simulink model "linmodel_eq1_discr_lqr"  (R2019a)
settings: Solver=VariableStepAuto  StartTime=0.0  StopTime=30  RelTol=1e-3
InitFcn:
  | lin_discr_model
undefined symbols (not defined in the file): A_eq1_d, B_eq1_d, C_eq1_d, K122, L, Ts
settings Model: Creator=jessi  LastModifiedBy=jessi

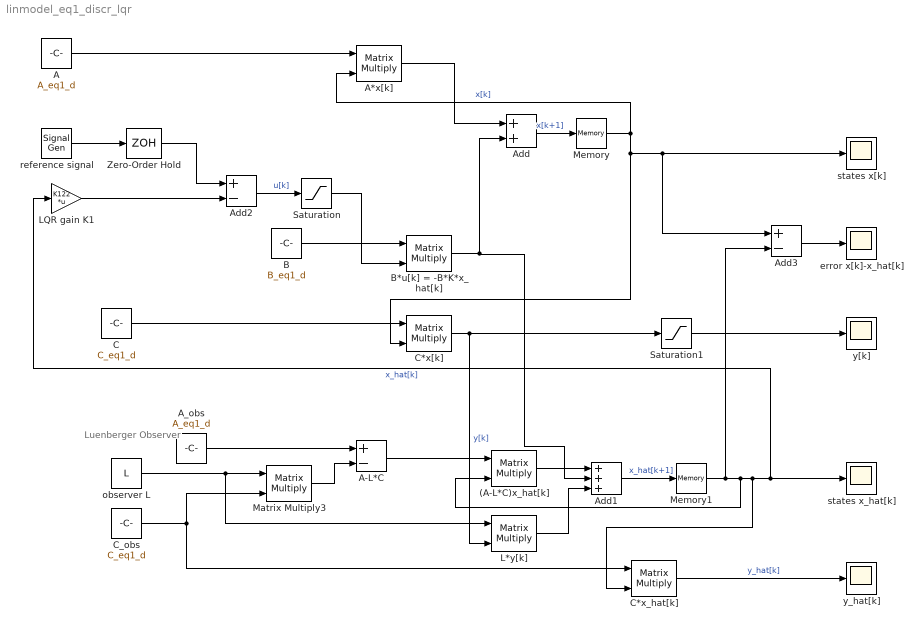
== system linmodel_eq1_discr_lqr ==
  note: Luenberger Observer
  (A-L*C)x_hat[k] : Product  Multiplication=Matrix(*)
  A : Constant  Value=A_eq1_d  SampleTime=Ts
  A*x[k] : Product  Multiplication=Matrix(*)
  A-L*C : Sum  Inputs=+-
  A_obs : Constant  Value=A_eq1_d
  Add : Sum
  Add1 : Sum  Inputs=+++
  Add2 : Sum  Inputs=+-
  Add3 : Sum  Inputs=+-
  B : Constant  Value=B_eq1_d  SampleTime=Ts
  B*u[k] = -B*K*x_hat[k] : Product  Multiplication=Matrix(*)
  C : Constant  Value=C_eq1_d  SampleTime=Ts
  C*x[k] : Product  Multiplication=Matrix(*)
  C*x_hat[k] : Product  Multiplication=Matrix(*)
  C_obs : Constant  Value=C_eq1_d
  L*y[k] : Product  Multiplication=Matrix(*)
  LQR gain K1 : Gain  Gain=K122  Multiplication=Matrix(K*u)
  Matrix Multiply3 : Product  Multiplication=Matrix(*)
  Memory : Memory  InitialCondition=[pi;0;0;0]
  Memory1 : Memory  InitialCondition=[pi; 0;0;0]
  Saturation : Saturate  UpperLimit=1  LowerLimit=-1
  Saturation1 : Saturate  UpperLimit=2*pi  LowerLimit=-2*pi
  Zero-Order Hold : ZeroOrderHold  SampleTime=Ts
  error x[k]-x_hat[k] : Scope
  observer L : Constant  Value=L  SampleTime=Ts
  reference signal : SignalGenerator  WaveForm=square  Amplitude=-0.3
  states x[k] : Scope
  states x_hat[k] : Scope
  y[k] : Scope
  y_hat[k] : Scope
  wires:
  B/1 -> B*u[k] = -B*K*x_hat[k]/1
  A/1 -> A*x[k]/1
  A*x[k]/1 -> Add/1
  B*u[k] = -B*K*x_hat[k]/1 -> Add1/2, Add/2
  Memory/1 -> A*x[k]/2, Add3/1, states x[k]/1, C*x[k]/2  "x[k]"
  C/1 -> C*x[k]/1
  C*x[k]/1 -> L*y[k]/2, Saturation1/1  "y[k]"
  observer L/1 -> L*y[k]/1, Matrix Multiply3/1
  Matrix Multiply3/1 -> A-L*C/2
  A-L*C/1 -> (A-L*C)x_hat[k]/1
  (A-L*C)x_hat[k]/1 -> Add1/1
  L*y[k]/1 -> Add1/3
  Add1/1 -> Memory1/1  "x_hat[k+1]"
  Memory1/1 -> Add3/2, (A-L*C)x_hat[k]/2, C*x_hat[k]/2, LQR gain K1/1, states x_hat[k]/1  "x_hat[k]"
  C*x_hat[k]/1 -> y_hat[k]/1  "y_hat[k]"
  Add/1 -> Memory/1  "x[k+1]"
  Add2/1 -> Saturation/1  "u[k]"
  Saturation/1 -> B*u[k] = -B*K*x_hat[k]/2
  Saturation1/1 -> y[k]/1
  Zero-Order Hold/1 -> Add2/1
  reference signal/1 -> Zero-Order Hold/1
  LQR gain K1/1 -> Add2/2
  Add3/1 -> error x[k]-x_hat[k]/1
  A_obs/1 -> A-L*C/1
  C_obs/1 -> C*x_hat[k]/1, Matrix Multiply3/2
